simulink model "k1visbsp_modal"  (Simulink 8.6)
settings: Solver=ode45  StartTime=0.0  StopTime=10.0  RelTol=1e-3
libraries: cdsIPCx x24, cdsEpicsOut x4, TYPEB_MASTER x3, cdsCDI64 x3, cdsCDO64 x3, dac x2, cdsAdcx0 x1, VIS_LIB x1, cdsParameters x1
settings Model: Creator=controls  LastModifiedBy=controls
settings DataIOCC: SignalLoggingSaveFormat=Dataset
settings OptimizationCC: ExpressionDepthLimit=128
settings DebuggingCC: UnderspecifiedInitializationDetection=Simplified  MergeDetectMultiDrivingBlocksExec=error  SolverPrmCheckMsg=none  FcnCallInpInsideContextMsg=EnableAllAsError  StateNameClashWarn=none
settings GRTTargetCC: CombineOutputUpdateFcns=on  GRTInterface=off

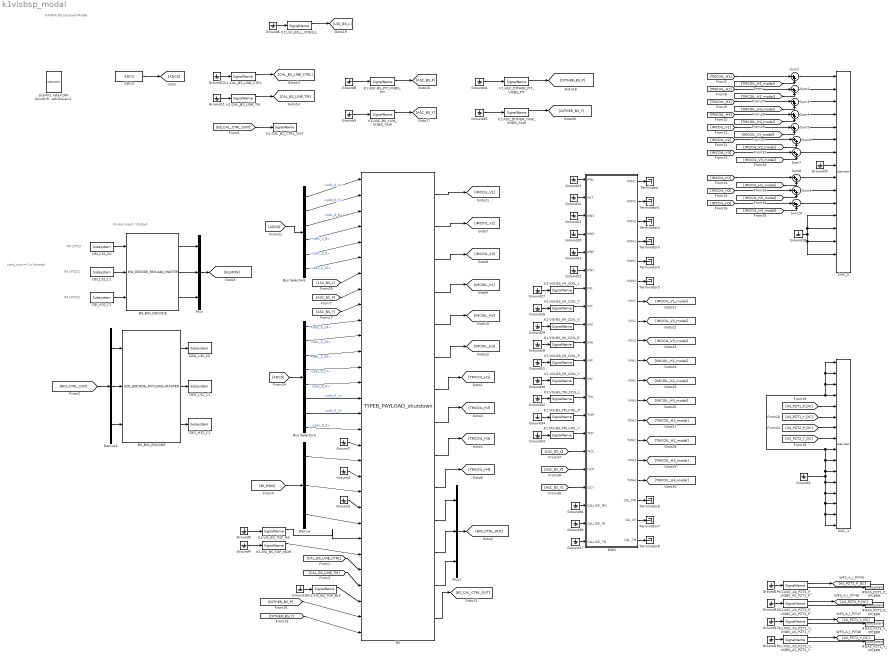
== system k1visbsp_modal ==
  note: KAGRA BS payload Model
  note: TM LPCD
  note: Binary Input / Output
  note: card_num=1 is Unused
  note: IM LPCD1
  note: IM LPCD2
  ADC0 : cdsAdcx0/ADC0  Tag=cdsAdc  Description=|
      | type-GSC_16AI64SSA
      | card_num=0
      settings: AttributesFormatString=%<Description>\n%<Tag>
  BS : TYPEB_MASTER/TYPEB_PAYLOAD_shutdown
  BS_BIO_DECODE : TYPEB_MASTER/BIO_DECODE_PAYLOAD_MASTER
  BS_BIO_ENCODE : TYPEB_MASTER/BIO_ENCODE_PAYLOAD_MASTER
  Bus Selector3 : BusSelector  Description=ADC Selector  OutputSignals=adc_0_24,adc_0_25,adc_0_26,adc_0_27,adc_0_0,adc_0_1,adc_0_2,adc_0_3
      settings: AttributesFormatString=%<Description>
  Bus Selector6 : BusSelector  Description=ADC Selector  OutputSignals=adc_0_4,adc_0_5,adc_0_6,adc_0_8,adc_0_9,adc_0_10
      settings: AttributesFormatString=%<Description>
  CBI_H32_C1 : cdsCDI64/Subsystem  Tag=cdsCDI64  Description=card_num=3
      settings: AttributesFormatString=%<Tag>\n%<Description>
  CBI_L32_C0 : cdsCDI64/Subsystem  Tag=cdsCDI64  Description=card_num=0
      settings: AttributesFormatString=%<Tag>\n%<Description>
  CBI_L32_C1 : cdsCDI64/Subsystem  Tag=cdsCDI64  Description=card_num=2
      settings: AttributesFormatString=%<Tag>\n%<Description>
  CBO_H32_C1 : cdsCDO64/Subsystem  Tag=cdsCDO64  Description=card_num=3
      settings: AttributesFormatString=%<Tag>\n%<Description>
  CBO_L32_C0 : cdsCDO64/Subsystem  Tag=cdsCDO64  Description=card_num=0
      settings: AttributesFormatString=%<Tag>\n%<Description>
  CBO_L32_C1 : cdsCDO64/Subsystem  Tag=cdsCDO64  Description=card_num=2
      settings: AttributesFormatString=%<Tag>\n%<Description>
  DAC_0 : dac/Subsystem  Description=|
      | type=GSC_16AO16,
      | card_num=0
      settings: AttributesFormatString=%<Description>
  DAC_1 : dac/Subsystem  Description=|
      | type=GSC_16AO16,
      | card_num=1
      settings: AttributesFormatString=%<Description>
  Demux : Demux  Outputs=3
  Demux1 : Demux  Outputs=3
  Ground{1..38} (38 alike) : Ground
  IFOAS_PZT1_P_IPCERR : cdsEpicsOut/Subsystem  Tag=cdsEpicsOutput  Description=|
      | Purpose:                                          
      | Output a FE signal to an EPICS channel.           
      |                                                   
      | Operation:                                        
      | Takes input value and passes it to EPICS record.  
      |                                                   
      | Usage:                                            
      | Name the part with the desired EPICS rrecord name.
      settings: AttributesFormatString=%<Tag>
  IFOAS_PZT1_Y_IPCERR : cdsEpicsOut/Subsystem  Tag=cdsEpicsOutput  Description=|
      | Purpose:                                          
      | Output a FE signal to an EPICS channel.           
      |                                                   
      | Operation:                                        
      | Takes input value and passes it to EPICS record.  
      |                                                   
      | Usage:                                            
      | Name the part with the desired EPICS rrecord name.
      settings: AttributesFormatString=%<Tag>
  IFOAS_PZT2_P_IPCERR : cdsEpicsOut/Subsystem  Tag=cdsEpicsOutput  Description=|
      | Purpose:                                          
      | Output a FE signal to an EPICS channel.           
      |                                                   
      | Operation:                                        
      | Takes input value and passes it to EPICS record.  
      |                                                   
      | Usage:                                            
      | Name the part with the desired EPICS rrecord name.
      settings: AttributesFormatString=%<Tag>
  IFOAS_PZT2_Y_IPCERR : cdsEpicsOut/Subsystem  Tag=cdsEpicsOutput  Description=|
      | Purpose:                                          
      | Output a FE signal to an EPICS channel.           
      |                                                   
      | Operation:                                        
      | Takes input value and passes it to EPICS record.  
      |                                                   
      | Usage:                                            
      | Name the part with the desired EPICS rrecord name.
      settings: AttributesFormatString=%<Tag>
  K1:ASC-BS_PIT_VISBS_PIT : cdsIPCx/SignalName  Tag=cdsIPCx_PCIE  Description=Inter-Process Communication via PCI Express network.
      settings: AttributesFormatString=%<Tag>
  K1:ASC-BS_YAW_VISBS_YAW : cdsIPCx/SignalName  Tag=cdsIPCx_PCIE  Description=Inter-Process Communication via PCI Express network.
      settings: AttributesFormatString=%<Tag>
  K1:ASC_AS_PZT1_P_VISBS_AS_PZT1_P : cdsIPCx/SignalName  Tag=cdsIPCx_PCIE  Description=Inter-Process Communication via PCI Express network.
      settings: AttributesFormatString=%<Tag>
  K1:ASC_AS_PZT1_Y_VISBS_AS_PZT1_Y : cdsIPCx/SignalName  Tag=cdsIPCx_PCIE  Description=Inter-Process Communication via PCI Express network.
      settings: AttributesFormatString=%<Tag>
  K1:ASC_AS_PZT2_P_VISBS_AS_PZT2_P : cdsIPCx/SignalName  Tag=cdsIPCx_PCIE  Description=Inter-Process Communication via PCI Express network.
      settings: AttributesFormatString=%<Tag>
  K1:ASC_AS_PZT2_Y_VISBS_AS_PZT2_Y : cdsIPCx/SignalName  Tag=cdsIPCx_PCIE  Description=Inter-Process Communication via PCI Express network.
      settings: AttributesFormatString=%<Tag>
  K1:ASC_DITHER_PIT_VISBS_PIT : cdsIPCx/SignalName  Tag=cdsIPCx_PCIE  Description=Inter-Process Communication via PCI Express network.
      settings: AttributesFormatString=%<Tag>
  K1:ASC_DITHER_YAW_VISBS_YAW : cdsIPCx/SignalName  Tag=cdsIPCx_PCIE  Description=Inter-Process Communication via PCI Express network.
      settings: AttributesFormatString=%<Tag>
  K1:CAL_BS_CTRL_OUT : cdsIPCx/SignalName  Tag=cdsIPCx_PCIE  Description=Inter-Process Communication via PCI Express network.
      settings: AttributesFormatString=%<Tag>
  K1:CAL_BS_LINE_CTRL : cdsIPCx/SignalName  Tag=cdsIPCx_PCIE  Description=Inter-Process Communication via PCI Express network.
      settings: AttributesFormatString=%<Tag>
  K1:CAL_BS_LINE_TM : cdsIPCx/SignalName  Tag=cdsIPCx_PCIE  Description=Inter-Process Communication via PCI Express network.
      settings: AttributesFormatString=%<Tag>
  K1:LSC_BS_L_VISBS_L : cdsIPCx/SignalName  Tag=cdsIPCx_PCIE  Description=Inter-Process Communication via PCI Express network.
      settings: AttributesFormatString=%<Tag>
  K1:VIS-BS_IM_COIL_L : cdsIPCx/SignalName  Tag=cdsIPCx_SHMEM  Description=Inter-Process Communication via Shared memory.
      settings: AttributesFormatString=%<Tag>
  K1:VIS-BS_IM_COIL_P : cdsIPCx/SignalName  Tag=cdsIPCx_SHMEM  Description=Inter-Process Communication via Shared memory.
      settings: AttributesFormatString=%<Tag>
  K1:VIS-BS_IM_COIL_R : cdsIPCx/SignalName  Tag=cdsIPCx_SHMEM  Description=Inter-Process Communication via Shared memory.
      settings: AttributesFormatString=%<Tag>
  K1:VIS-BS_IM_COIL_T : cdsIPCx/SignalName  Tag=cdsIPCx_SHMEM  Description=Inter-Process Communication via Shared memory.
      settings: AttributesFormatString=%<Tag>
  K1:VIS-BS_IM_COIL_V : cdsIPCx/SignalName  Tag=cdsIPCx_SHMEM  Description=Inter-Process Communication via Shared memory.
      settings: AttributesFormatString=%<Tag>
  K1:VIS-BS_IM_COIL_Y : cdsIPCx/SignalName  Tag=cdsIPCx_SHMEM  Description=Inter-Process Communication via Shared memory.
      settings: AttributesFormatString=%<Tag>
  K1:VIS-BS_TM_COIL_L : cdsIPCx/SignalName  Tag=cdsIPCx_SHMEM  Description=Inter-Process Communication via Shared memory.
      settings: AttributesFormatString=%<Tag>
  K1:VIS-BS_TM_COIL_P : cdsIPCx/SignalName  Tag=cdsIPCx_SHMEM  Description=Inter-Process Communication via Shared memory.
      settings: AttributesFormatString=%<Tag>
  K1:VIS-BS_TM_COIL_Y : cdsIPCx/SignalName  Tag=cdsIPCx_SHMEM  Description=Inter-Process Communication via Shared memory.
      settings: AttributesFormatString=%<Tag>
  K1:VIS_BS_TOP_BLF : cdsIPCx/SignalName  Tag=cdsIPCx_SHMEM  Description=Inter-Process Communication via Shared memory.
      settings: AttributesFormatString=%<Tag>
  K1:VIS_BS_TOP_MS : cdsIPCx/SignalName  Tag=cdsIPCx_SHMEM  Description=Inter-Process Communication via Shared memory.
      settings: AttributesFormatString=%<Tag>
  K1:VIS_BS_TOP_WDR : cdsIPCx/SignalName  Tag=cdsIPCx_SHMEM  Description=Inter-Process Communication via Shared memory.
      settings: AttributesFormatString=%<Tag>
  MOD : Subsystem  Tag=top_names
  Mux : Mux  Inputs=3
  Mux1 : Mux  Inputs=3
  Sum{1..10} (10 alike) : Sum  Inputs=|++
  Terminator{,1..8} (9 alike) : Terminator
  site=K1 rate=16K dcuid=92 host=k1bs specific_cpu=5 adcSlave=1 : cdsParameters/Subsystem  Tag=cdsParameters  Description=|
      | Purpose:                                                                                                                                                                                                                                
      | Provide system parameters to the FE code generator to properly configure the generated EPICS names, rep rate of the FE controller, and the Data Acquisition node ID for proper storage of data from this FE controller.                 
      |                                                                                                                                                                                                                                         
      | Useage:                                                                                                                                                                                                                                 
      | The part NAME field is used to identify the FE parameters. It must be of the form:                                                                                                                                                      
      | site=                                                                                                                                                                                                                                   
      | rate=                                                                                                                                                                                                                                   
      | dcuid=                                                                                                                                                                                                                                  
      |                                                                                                                                                                                                                                         
      | Where:                                                                                                                                                                                                                                  
      | site= argument may be H1, H2, L1, M1, G1, either as a single argument or multiple, for example site=H1,H2. These are the only names allowed. These will become the first two characters of all EPICS and signal names (for example G1:).
      |                                                                                                                                                                                                                                         
      | rate= may be 2K, 16K, 32K, or 64K                                                                                                                                                                                                       
      |                                                                                                                                                                                                                                         
      | dcuid= is site specific ie it must be unique at each site.
      settings: AttributesFormatString=%<Tag>
  wires:
  ADC0/1 -> [ADC0]
  [ADC0] -> Bus Selector6/1
  BS/10 -> [TMCOIL_H4]
  BS/9 -> [TMCOIL_H3]
  BS/8 -> [TMCOIL_H2]
  BS/7 -> [TMCOIL_H1]
  BS/1 -> [IMCOIL_V1]
  BS/2 -> [IMCOIL_V2]
  BS/3 -> [IMCOIL_V3]
  BS/4 -> [IMCOIL_H1]
  BS/5 -> [IMCOIL_H2]
  BS/6 -> [IMCOIL_H3]
  Ground18/1 -> DAC_0/12, DAC_0/13, DAC_0/15, DAC_0/14
  Bus Selector6/1 -> BS/1  "<adc_0_4>"
  Bus Selector6/2 -> BS/2  "<adc_0_5>"
  Bus Selector6/3 -> BS/3  "<adc_0_6>"
  [TMCOIL_H1] -> Sum1/1
  [IMCOIL_V1] -> Sum5/1
  Bus Selector6/4 -> BS/4  "<adc_0_8>"
  Bus Selector6/5 -> BS/5  "<adc_0_9>"
  Bus Selector6/6 -> BS/6  "<adc_0_10>"
  [LSC_BS_L] -> BS/7
  [ADC0] -> Bus Selector3/1
  Bus Selector3/1 -> BS/10  "<adc_0_24>"
  Bus Selector3/2 -> BS/11  "<adc_0_25>"
  Bus Selector3/3 -> BS/12  "<adc_0_26>"
  Bus Selector3/4 -> BS/13  "<adc_0_27>"
  BS_BIO_ENCODE/3 -> CBO_H32_C1/1
  BS_BIO_ENCODE/2 -> CBO_L32_C1/1
  CBI_L32_C1/1 -> BS_BIO_DECODE/2
  CBI_H32_C1/1 -> BS_BIO_DECODE/3
  BS_BIO_DECODE/2 -> Mux/2
  BS_BIO_DECODE/3 -> Mux/3
  BS_BIO_DECODE/1 -> Mux/1
  Mux/1 -> [BI_MON]
  Demux1/2 -> BS_BIO_ENCODE/2
  Demux1/3 -> BS_BIO_ENCODE/3
  Demux1/1 -> BS_BIO_ENCODE/1
  [BIO_CTRL_OUT] -> Demux1/1
  Mux1/1 -> [BIO_CTRL_OUT]
  [BI_MON] -> Demux/1
  Demux/1 -> BS/19
  Demux/2 -> BS/21
  Demux/3 -> BS/23
  Ground7/1 -> BS/18
  Ground1/1 -> BS/22
  Ground2/1 -> BS/20
  Ground4/1 -> K1:VIS_BS_TOP_WDR/1
  Ground5/1 -> K1:VIS_BS_TOP_MS/1
  K1:VIS_BS_TOP_WDR/1 -> BS/25
  K1:VIS_BS_TOP_MS/1 -> BS/24
  Ground10/1 -> K1:CAL_BS_LINE_CTRL/1
  K1:CAL_BS_LINE_CTRL/1 -> [CAL_BS_LINE_CTRL]
  Ground11/1 -> K1:CAL_BS_LINE_TM/1
  K1:CAL_BS_LINE_TM/1 -> [CAL_BS_LINE_TM]
  [CAL_BS_LINE_CTRL] -> BS/26
  [CAL_BS_LINE_TM] -> BS/27
  BS/14 -> [BS_CAL_CTRL_OUT]
  [BS_CAL_CTRL_OUT] -> K1:CAL_BS_CTRL_OUT/1
  Ground3/1 -> DAC_1/13, DAC_1/14, DAC_1/15, DAC_1/16, DAC_1/12, DAC_1/1, DAC_1/2, DAC_1/3, DAC_1/4, DAC_1/9, DAC_1/10, DAC_1/11
  Bus Selector3/5 -> BS/14  "<adc_0_0>"
  Bus Selector3/6 -> BS/15  "<adc_0_1>"
  Bus Selector3/7 -> BS/16  "<adc_0_2>"
  Bus Selector3/8 -> BS/17  "<adc_0_3>"
  [ASC_BS_P] -> BS/8
  [ASC_BS_Y] -> BS/9
  Ground16/1 -> K1:VIS_BS_TOP_BLF/1
  K1:VIS_BS_TOP_BLF/1 -> BS/28
  BS/11 -> Mux1/1
  BS/12 -> Mux1/2
  BS/13 -> Mux1/3
  [DITHER_BS_Y] -> BS/30
  K1:ASC_AS_PZT1_P_VISBS_AS_PZT1_P/2 -> IFOAS_PZT1_P_IPCERR/1
  K1:ASC_AS_PZT2_P_VISBS_AS_PZT2_P/2 -> IFOAS_PZT2_P_IPCERR/1
  K1:ASC_AS_PZT1_Y_VISBS_AS_PZT1_Y/2 -> IFOAS_PZT1_Y_IPCERR/1
  K1:ASC_AS_PZT2_Y_VISBS_AS_PZT2_Y/2 -> IFOAS_PZT2_Y_IPCERR/1
  K1:ASC_AS_PZT1_P_VISBS_AS_PZT1_P/1 -> [AS_PZT1_P_DC]
  K1:ASC_AS_PZT2_P_VISBS_AS_PZT2_P/1 -> [AS_PZT2_P_DC]
  K1:ASC_AS_PZT1_Y_VISBS_AS_PZT1_Y/1 -> [AS_PZT1_Y_DC]
  K1:ASC_AS_PZT2_Y_VISBS_AS_PZT2_Y/1 -> [AS_PZT2_Y_DC]
  Ground14/1 -> K1:ASC_AS_PZT1_P_VISBS_AS_PZT1_P/1
  Ground15/1 -> K1:ASC_AS_PZT2_P_VISBS_AS_PZT2_P/1
  Ground17/1 -> K1:ASC_AS_PZT1_Y_VISBS_AS_PZT1_Y/1
  Ground19/1 -> K1:ASC_AS_PZT2_Y_VISBS_AS_PZT2_Y/1
  [AS_PZT2_Y_DC] -> DAC_1/8
  [AS_PZT2_P_DC] -> DAC_1/7
  [AS_PZT1_Y_DC] -> DAC_1/6
  [AS_PZT1_P_DC] -> DAC_1/5
  Ground6/1 -> K1:LSC_BS_L_VISBS_L/1
  K1:LSC_BS_L_VISBS_L/1 -> [LSC_BS_L]
  Ground8/1 -> K1:ASC-BS_PIT_VISBS_PIT/1
  Ground9/1 -> K1:ASC-BS_YAW_VISBS_YAW/1
  Ground25/1 -> K1:ASC_DITHER_YAW_VISBS_YAW/1
  Ground24/1 -> K1:ASC_DITHER_PIT_VISBS_PIT/1
  [DITHER_BS_P] -> BS/29
  K1:ASC-BS_PIT_VISBS_PIT/1 -> [ASC_BS_P]
  K1:ASC-BS_YAW_VISBS_YAW/1 -> [ASC_BS_Y]
  K1:ASC_DITHER_PIT_VISBS_PIT/1 -> [DITHER_BS_P]
  K1:ASC_DITHER_YAW_VISBS_YAW/1 -> [DITHER_BS_Y]
  BS_BIO_ENCODE/1 -> CBO_L32_C0/1
  CBI_L32_C0/1 -> BS_BIO_DECODE/1
  Ground13/1 -> MOD/1(MNL)
  Ground12/1 -> MOD/2(MLT)
  Ground21/1 -> MOD/3(MNV)
  Ground20/1 -> MOD/4(MNR)
  Ground23/1 -> MOD/5(MNP)
  Ground22/1 -> MOD/6(MNY)
  K1:VIS-BS_IM_COIL_L/1 -> MOD/7(IML)
  K1:VIS-BS_IM_COIL_T/1 -> MOD/8(IMT)
  K1:VIS-BS_IM_COIL_V/1 -> MOD/9(IMV)
  K1:VIS-BS_IM_COIL_R/1 -> MOD/10(IMR)
  K1:VIS-BS_IM_COIL_P/1 -> MOD/11(IMP)
  K1:VIS-BS_IM_COIL_Y/1 -> MOD/12(IMY)
  K1:VIS-BS_TM_COIL_L/1 -> MOD/13(TML)
  K1:VIS-BS_TM_COIL_P/1 -> MOD/14(TMP)
  K1:VIS-BS_TM_COIL_Y/1 -> MOD/15(TMY)
  Ground27/1 -> K1:VIS-BS_IM_COIL_L/1
  Ground26/1 -> K1:VIS-BS_IM_COIL_T/1
  Ground29/1 -> K1:VIS-BS_IM_COIL_V/1
  Ground28/1 -> K1:VIS-BS_IM_COIL_R/1
  Ground31/1 -> K1:VIS-BS_IM_COIL_P/1
  Ground30/1 -> K1:VIS-BS_IM_COIL_Y/1
  Ground32/1 -> K1:VIS-BS_TM_COIL_L/1
  Ground34/1 -> K1:VIS-BS_TM_COIL_P/1
  Ground33/1 -> K1:VIS-BS_TM_COIL_Y/1
  MOD/1(MNV1) -> Terminator/1
  MOD/2(MNV2) -> Terminator1/1
  MOD/3(MNV3) -> Terminator2/1
  MOD/4(MNH1) -> Terminator3/1
  MOD/5(MNH2) -> Terminator4/1
  MOD/6(MNH3) -> Terminator5/1
  Ground35/1 -> DAC_0/8
  MOD/7(IMV1) -> [IMCOIL_V1_modal]
  MOD/8(IMV2) -> [IMCOIL_V2_modal]
  MOD/9(IMV3) -> [IMCOIL_V3_modal]
  MOD/10(IMH1) -> [IMCOIL_H1_modal]
  MOD/11(IMH2) -> [IMCOIL_H2_modal]
  MOD/12(IMH3) -> [IMCOIL_H3_modal]
  MOD/13(TMH1) -> [TMCOIL_H1_modal]
  MOD/14(TMH2) -> [TMCOIL_H2_modal]
  MOD/15(TMH3) -> [TMCOIL_H3_modal]
  MOD/16(TMH4) -> [TMCOIL_H4_modal]
  MOD/17(CAL_MN) -> Terminator6/1
  MOD/18(CAL_IM) -> Terminator7/1
  MOD/19(CAL_TM) -> Terminator8/1
  [TMCOIL_H1_modal] -> Sum1/2
  Sum1/1 -> DAC_0/1
  [TMCOIL_H2_modal] -> Sum2/2
  Sum2/1 -> DAC_0/2
  [TMCOIL_H2] -> Sum2/1
  [TMCOIL_H3_modal] -> Sum3/2
  Sum3/1 -> DAC_0/3
  [TMCOIL_H3] -> Sum3/1
  [TMCOIL_H4_modal] -> Sum4/2
  Sum4/1 -> DAC_0/4
  [TMCOIL_H4] -> Sum4/1
  [IMCOIL_V1_modal] -> Sum5/2
  Sum5/1 -> DAC_0/5
  [IMCOIL_V2_modal] -> Sum6/2
  Sum6/1 -> DAC_0/6
  [IMCOIL_V2] -> Sum6/1
  [IMCOIL_V3_modal] -> Sum7/2
  Sum7/1 -> DAC_0/7
  [IMCOIL_V3] -> Sum7/1
  [IMCOIL_H1_modal] -> Sum8/2
  Sum8/1 -> DAC_0/9
  [IMCOIL_H1] -> Sum8/1
  [IMCOIL_H2_modal] -> Sum9/2
  Sum9/1 -> DAC_0/10
  [IMCOIL_H2] -> Sum9/1
  [IMCOIL_H3_modal] -> Sum10/2
  Sum10/1 -> DAC_0/11
  [IMCOIL_H3] -> Sum10/1
  [LSC_BS_L] -> MOD/16(ISCL)
  [ASC_BS_P] -> MOD/17(ISCP)
  [ASC_BS_Y] -> MOD/18(ISCY)
  Ground36/1 -> MOD/19(CALLINE_MN)
  Ground38/1 -> MOD/20(CALLINE_IM)
  Ground37/1 -> MOD/21(CALLINE_TM)

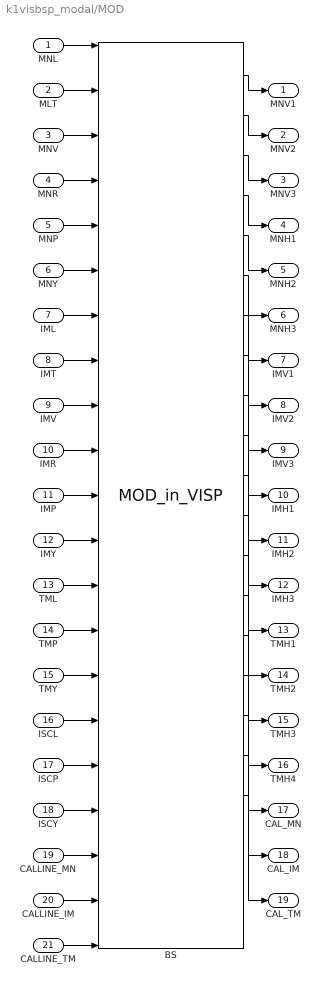
== system k1visbsp_modal/MOD ==
  MNL : Inport
  MLT : Inport  Port=2
  MNV : Inport  Port=3
  MNR : Inport  Port=4
  MNP : Inport  Port=5
  MNY : Inport  Port=6
  IML : Inport  Port=7
  IMT : Inport  Port=8
  IMV : Inport  Port=9
  IMR : Inport  Port=10
  IMP : Inport  Port=11
  IMY : Inport  Port=12
  TML : Inport  Port=13
  TMP : Inport  Port=14
  TMY : Inport  Port=15
  ISCL : Inport  Port=16
  ISCP : Inport  Port=17
  ISCY : Inport  Port=18
  CALLINE_MN : Inport  Port=19
  CALLINE_IM : Inport  Port=20
  CALLINE_TM : Inport  Port=21
  BS : VIS_LIB/MODAL/MOD_in_VISP  Tag=top_names
  MNV1 : Outport
  MNV2 : Outport  Port=2
  MNV3 : Outport  Port=3
  MNH1 : Outport  Port=4
  MNH2 : Outport  Port=5
  MNH3 : Outport  Port=6
  IMV1 : Outport  Port=7
  IMV2 : Outport  Port=8
  IMV3 : Outport  Port=9
  IMH1 : Outport  Port=10
  IMH2 : Outport  Port=11
  IMH3 : Outport  Port=12
  TMH1 : Outport  Port=13
  TMH2 : Outport  Port=14
  TMH3 : Outport  Port=15
  TMH4 : Outport  Port=16
  CAL_MN : Outport  Port=17
  CAL_IM : Outport  Port=18
  CAL_TM : Outport  Port=19
  wires:
  MNL/1 -> BS/1
  TMY/1 -> BS/15
  MLT/1 -> BS/2
  MNV/1 -> BS/3
  MNR/1 -> BS/4
  MNP/1 -> BS/5
  MNY/1 -> BS/6
  IML/1 -> BS/7
  IMT/1 -> BS/8
  IMV/1 -> BS/9
  IMR/1 -> BS/10
  IMP/1 -> BS/11
  IMY/1 -> BS/12
  TML/1 -> BS/13
  TMP/1 -> BS/14
  BS/1 -> MNV1/1
  BS/16 -> TMH4/1
  BS/2 -> MNV2/1
  BS/3 -> MNV3/1
  BS/4 -> MNH1/1
  BS/5 -> MNH2/1
  BS/6 -> MNH3/1
  BS/7 -> IMV1/1
  BS/8 -> IMV2/1
  BS/9 -> IMV3/1
  BS/10 -> IMH1/1
  BS/11 -> IMH2/1
  BS/12 -> IMH3/1
  BS/13 -> TMH1/1
  BS/14 -> TMH2/1
  BS/15 -> TMH3/1
  ISCL/1 -> BS/16
  CALLINE_TM/1 -> BS/21
  CALLINE_IM/1 -> BS/20
  CALLINE_MN/1 -> BS/19
  ISCP/1 -> BS/17
  ISCY/1 -> BS/18
  BS/17 -> CAL_MN/1
  BS/18 -> CAL_IM/1
  BS/19 -> CAL_TM/1
